simulink model "ModulateurSigmaDelta"  (R2023a)
settings: Solver=ode3  StartTime=0.0  StopTime=Tsim  FixedStep=TsR  RelTol=1e-3  EnableMultiTasking=on
undefined symbols (not defined in the file or in its folder): nu0
settings Model: ExtModeTrigMode=oneshot  Creator=gscorlet  LastModifiedBy=arthur.perodou
settings SolverCC: AlgebraicLoopSolver=TrustRegion
settings DataIOCC: SaveFormat=Array  SignalLoggingSaveFormat=ModelDataLogs  ReturnWorkspaceOutputs=off
settings OptimizationCC: BlockReduction=off  BooleanDataType=off  ReuseModelBlockBuffer=off  ExpressionDepthLimit=2147483647  LifeSpan=inf
settings DebuggingCC: SaveWithParameterizedLinksMsg=none  UnderspecifiedInitializationDetection=Classic  MergeDetectMultiDrivingBlocksExec=none  SignalResolutionControl=TryResolveAllWithWarning  MultiTaskDSMMsg=warning  MultiTaskCondExecSysMsg=none  FcnCallInpInsideContextMsg=warning  UnconnectedInputMsg=warning  UnconnectedOutputMsg=warning  UnconnectedLineMsg=warning  StateNameClashWarn=warning  SFUnexpectedBacktrackingDiag=warning  SFNoUnconditionalDefaultTransitionDiag=warning  SFExecutionAtInitializationDiag=none  ArithmeticOperatorsInVariantConditions=warning
settings HardwareCC: ProdBitPerPointer=32  ProdBitPerSizeT=32  ProdBitPerPtrDiffT=32  ProdLargestAtomicFloat=None  ProdIntDivRoundTo=Undefined  ProdEndianess=Unspecified  ProdWordSize=32  ProdHWDeviceType=32-bit Generic  TargetUnknown=on
settings ModelReferenceCC: PropagateSignalLabelsOutOfModel=off
settings SFSimCC: SimUseLocalCustomCode=off  CustomCodeUndefinedFunction=UseInterfaceOnly
settings RTWCC: RTWUseLocalCustomCode=off
settings CodeAppCC: StateflowObjectComments=on
settings GRTTargetCC: TargetLangStandard=C89/C90 (ANSI)  CombineOutputUpdateFcns=off  GRTInterface=on
settings ConfigComp: CovMetricSettings=dw  CovSaveCumulativeToWorkspaceVar=on  CovSaveSingleToWorkspaceVar=on  CovExternalEMLEnable=off  CovBoundaryAbsTol=1.0e-5

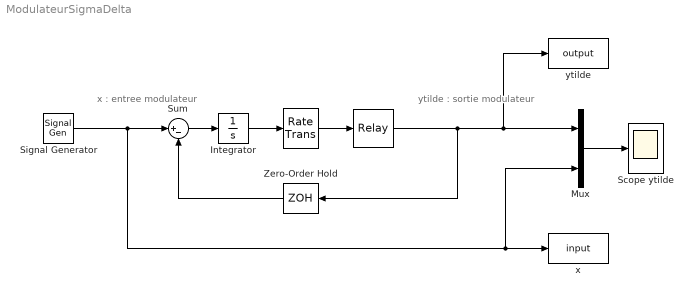
== system ModulateurSigmaDelta ==
  note: x : entree
      | modulateur
  note: ytilde : sortie
      | modulateur
  " " : Relay  OffSwitchValue=-eps  OffOutputValue=-1
  "   " : RateTransition  OutPortSampleTime=TsR
  Integrator : Integrator
  Mux : Mux  Inputs=2
  Scope ytilde : Scope
  Signal Generator : SignalGenerator  Frequency=nu0
  Sum : Sum  Inputs=|+-  InputSameDT=on  SaturateOnIntegerOverflow=on  OutDataTypeStr=Inherit: Same as first input
  Zero-Order Hold : ZeroOrderHold  SampleTime=-1
  x : ToWorkspace  VariableName=input  SaveFormat=Timeseries  SampleTime=-1
  ytilde : ToWorkspace  VariableName=output  SaveFormat=Timeseries  SampleTime=-1
  wires:
  Integrator/1 -> "   "/1
  Sum/1 -> Integrator/1
  Signal Generator/1 -> Sum/1, x/1, Mux/2
  Mux/1 -> Scope ytilde/1
  "   "/1 -> " "/1
  " "/1 -> ytilde/1, Mux/1, Zero-Order Hold/1
  Zero-Order Hold/1 -> Sum/2
